simulink model "Control_5_States_feedback"  (R2017b)
settings: Solver=VariableStepAuto  StartTime=0.0  StopTime=TMax  RelTol=1e-3
values from neighbouring files (symbols this model uses):
  alpha = exp(-2*pi*DT*fc)    [lqr5.m]
  DT = 0.01    [lqr5.m]
  G = -K    [lqr5.m]
  PC_MaxPit = 1.570796    [lqr5.m]
  PC_MaxRat = 0.1396263    [lqr5.m]
  PC_MinPit = 0.0    (= 0)    [lqr5.m]
  ref_DrTr = Avgxop(DrTr)    [lqr5.m]
  ref_DrTrdot = Avgxop(DrTrdot)    [lqr5.m]
  ref_pitch = 7.16347E-02    (= 0.0716347)    [lqr5.m]
  ref_rot = Avgxop(rot_speed)    [lqr5.m]
  ref_symfp = (Avgxop(FP1)+Avgxop(FP2)+Avgxop(FP3))/3    [lqr5.m]
  ref_symfpdot = (Avgxop(FP1s)+Avgxop(FP2s)+Avgxop(FP3s))/3    [lqr5.m]
undefined symbols (not defined in the file or in its folder): OutList, strmatch
settings Model: Creator=Avell 1513  LastModifiedBy=Avell 1513

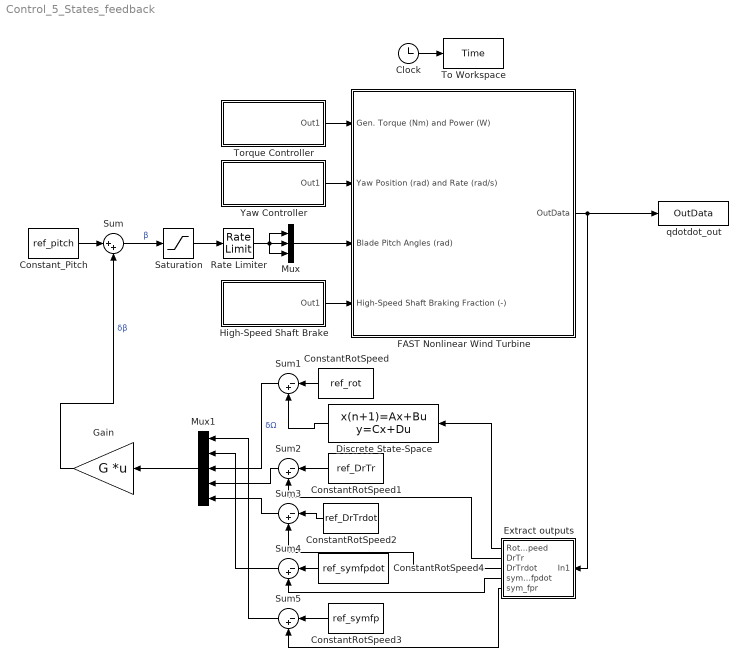
== system Control_5_States_feedback ==
  Clock : Clock
  ConstantRotSpeed : Constant  Value=ref_rot
  ConstantRotSpeed1 : Constant  Value=ref_DrTr
  ConstantRotSpeed2 : Constant  Value=ref_DrTrdot
  ConstantRotSpeed3 : Constant  Value=ref_symfp
  ConstantRotSpeed4 : Constant  Value=ref_symfpdot
  Constant_Pitch : Constant  Value=ref_pitch
  Discrete State-Space : DiscreteStateSpace  A=alpha  B=1-alpha  C=alpha  D=1-alpha  InitialCondition=ref_rot  SampleTime=DT
  Extract outputs : Subsystem
  FAST Nonlinear Wind Turbine : Subsystem  mask(FAST Nonlinear Wind Turbine){}
      mask help: This block contains the FAST S-Function.
      mask init:
      | clear FAST_SFunc
  Gain : Gain  Gain=G  Multiplication=Matrix(K*u)
  High-Speed Shaft Brake : Subsystem
  Mux : Mux  Inputs=3
  Mux1 : Mux  Inputs=5
  Rate Limiter : RateLimiter  RisingSlewLimit=PC_MaxRat  FallingSlewLimit=-PC_MaxRat  SampleTimeMode=inherited
  Saturation : Saturate  UpperLimit=PC_MaxPit  LowerLimit=PC_MinPit
  Sum : Sum  Inputs=|++
  Sum{1..5} (5 alike) : Sum  Inputs=|-+
  To Workspace : ToWorkspace  VariableName=Time  SampleTime=-1
  Torque Controller : Subsystem
  Yaw Controller : Subsystem
  qdotdot_out : ToWorkspace  VariableName=OutData  SampleTime=-1
  wires:
  Gain/1 -> Sum/2  "δβ"
  Yaw Controller/1(Out1) -> FAST Nonlinear Wind Turbine/2(Yaw Position (rad) and Rate (rad/s))
  High-Speed Shaft Brake/1(Out1) -> FAST Nonlinear Wind Turbine/4(High-Speed Shaft Braking Fraction (-))
  Discrete State-Space/1 -> Sum1/2
  Constant_Pitch/1 -> Sum/1
  FAST Nonlinear Wind Turbine/1(OutData) -> qdotdot_out/1, Extract outputs/1(In1)
  Saturation/1 -> Rate Limiter/1
  Clock/1 -> To Workspace/1
  Sum/1 -> Saturation/1  "β"
  Rate Limiter/1 -> Mux/1, Mux/3, Mux/2
  ConstantRotSpeed/1 -> Sum1/1
  Mux/1 -> FAST Nonlinear Wind Turbine/3(Blade Pitch Angles (rad))
  Torque Controller/1(Out1) -> FAST Nonlinear Wind Turbine/1(Gen. Torque (Nm) and Power (W))
  Sum1/1 -> Mux1/3  "δΩ"
  Extract outputs/1(Rot_speed) -> Discrete State-Space/1
  ConstantRotSpeed2/1 -> Sum3/1
  ConstantRotSpeed1/1 -> Sum2/1
  Extract outputs/5(sym_fpr) -> Sum5/2
  Extract outputs/4(sym_fpdot) -> Sum4/2
  Extract outputs/3(DrTrdot) -> Sum3/2
  Extract outputs/2(DrTr) -> Sum2/2
  Mux1/1 -> Gain/1
  Sum2/1 -> Mux1/4
  Sum3/1 -> Mux1/5
  ConstantRotSpeed4/1 -> Sum4/1
  ConstantRotSpeed3/1 -> Sum5/1
  Sum4/1 -> Mux1/2
  Sum5/1 -> Mux1/1

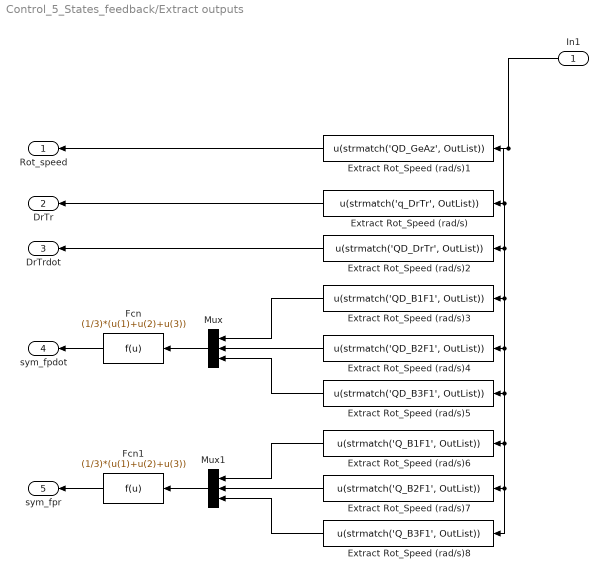
== system Control_5_States_feedback/Extract outputs ==
  In1 : Inport
  Extract Rot_Speed (rad/s) : Fcn  Expr=u(strmatch('q_DrTr', OutList))
  Extract Rot_Speed (rad/s)1 : Fcn  Expr=u(strmatch('QD_GeAz', OutList))
  Extract Rot_Speed (rad/s)2 : Fcn  Expr=u(strmatch('QD_DrTr', OutList))
  Extract Rot_Speed (rad/s)3 : Fcn  Expr=u(strmatch('QD_B1F1', OutList))
  Extract Rot_Speed (rad/s)4 : Fcn  Expr=u(strmatch('QD_B2F1', OutList))
  Extract Rot_Speed (rad/s)5 : Fcn  Expr=u(strmatch('QD_B3F1', OutList))
  Extract Rot_Speed (rad/s)6 : Fcn  Expr=u(strmatch('Q_B1F1', OutList))
  Extract Rot_Speed (rad/s)7 : Fcn  Expr=u(strmatch('Q_B2F1', OutList))
  Extract Rot_Speed (rad/s)8 : Fcn  Expr=u(strmatch('Q_B3F1', OutList))
  Fcn : Fcn  Expr=(1/3)*(u(1)+u(2)+u(3))
  Fcn1 : Fcn  Expr=(1/3)*(u(1)+u(2)+u(3))
  Mux : Mux  Inputs=3
  Mux1 : Mux  Inputs=3
  Rot_speed : Outport
  DrTr : Outport  Port=2
  DrTrdot : Outport  Port=3
  sym_fpdot : Outport  Port=4
  sym_fpr : Outport  Port=5
  wires:
  Extract Rot_Speed (rad/s)1/1 -> Rot_speed/1
  Extract Rot_Speed (rad/s)2/1 -> DrTrdot/1
  Extract Rot_Speed (rad/s)/1 -> DrTr/1
  In1/1 -> Extract Rot_Speed (rad/s)2/1, Extract Rot_Speed (rad/s)3/1, Extract Rot_Speed (rad/s)4/1, Extract Rot_Speed (rad/s)6/1, Extract Rot_Speed (rad/s)7/1, Extract Rot_Speed (rad/s)8/1, Extract Rot_Speed (rad/s)5/1, Extract Rot_Speed (rad/s)/1, Extract Rot_Speed (rad/s)1/1
  Fcn/1 -> sym_fpdot/1
  Fcn1/1 -> sym_fpr/1
  Mux1/1 -> Fcn1/1
  Mux/1 -> Fcn/1
  Extract Rot_Speed (rad/s)3/1 -> Mux/1
  Extract Rot_Speed (rad/s)4/1 -> Mux/2
  Extract Rot_Speed (rad/s)5/1 -> Mux/3
  Extract Rot_Speed (rad/s)6/1 -> Mux1/1
  Extract Rot_Speed (rad/s)7/1 -> Mux1/2
  Extract Rot_Speed (rad/s)8/1 -> Mux1/3

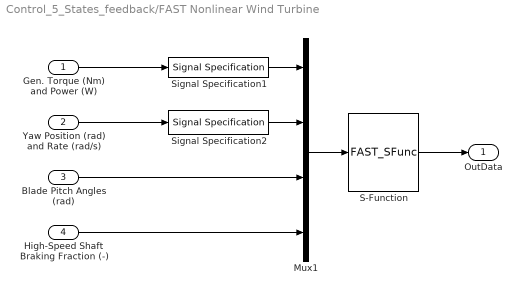
== system Control_5_States_feedback/FAST Nonlinear Wind Turbine ==
  Gen. Torque (Nm) and Power (W) : Inport
  Yaw Position (rad) and Rate (rad/s) : Inport  Port=2
  Blade Pitch Angles (rad) : Inport  Port=3
  High-Speed Shaft Braking Fraction (-) : Inport  Port=4
  Mux1 : Mux
  S-Function : S-Function  FunctionName=FAST_SFunc  Parameters=FAST_InputFileName, TMax, 0  SFunctionDeploymentMode=off  EnableBusSupport=off
  Signal Specification1 : SignalSpecification  OutDataTypeStr=double  Dimensions=2
  Signal Specification2 : SignalSpecification  OutDataTypeStr=double  Dimensions=2
  OutData : Outport
  wires:
  Gen. Torque (Nm) and Power (W)/1 -> Signal Specification1/1
  S-Function/1 -> OutData/1
  Mux1/1 -> S-Function/1
  Blade Pitch Angles (rad)/1 -> Mux1/3
  Yaw Position (rad) and Rate (rad/s)/1 -> Signal Specification2/1
  Signal Specification1/1 -> Mux1/1
  Signal Specification2/1 -> Mux1/2
  High-Speed Shaft Braking Fraction (-)/1 -> Mux1/4

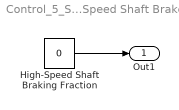
== system Control_5_States_feedback/High-Speed Shaft Brake ==
  High-Speed Shaft Braking Fraction : Constant  Value=0
  Out1 : Outport
  wires:
  High-Speed Shaft Braking Fraction/1 -> Out1/1

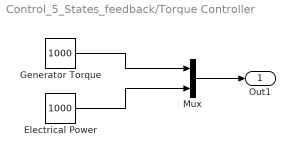
== system Control_5_States_feedback/Torque Controller ==
  Electrical Power : Constant  Value=1000
  Generator Torque : Constant  Value=1000
  Mux : Mux  Inputs=2
  Out1 : Outport
  wires:
  Mux/1 -> Out1/1
  Generator Torque/1 -> Mux/1
  Electrical Power/1 -> Mux/2

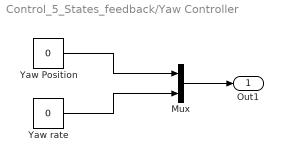
== system Control_5_States_feedback/Yaw Controller ==
  Mux : Mux  Inputs=2
  Yaw Position : Constant  Value=0
  Yaw rate : Constant  Value=0
  Out1 : Outport
  wires:
  Mux/1 -> Out1/1
  Yaw Position/1 -> Mux/1
  Yaw rate/1 -> Mux/2
